simulink model "gridv1"  (R2021a)
settings: Solver=VariableStepAuto  StartTime=0.0  StopTime=inf  RelTol=1e-3
libraries: spsThreePhaseBreakerLib x12, spsMosfetLib x12, spsThreePhaseSeriesRLCLoadLib x10, spsMeanLib x6, pid_lib x5, simulink x4, spsPLL3phLib x4, spsThreePhaseVIMeasurementLib x4, spsAsynchronousMachineSIUnitsLib x2, spsDCVoltageSourceLib x2, spsFourierLib x2, spsGroundLib x2
(part 2 of 2)

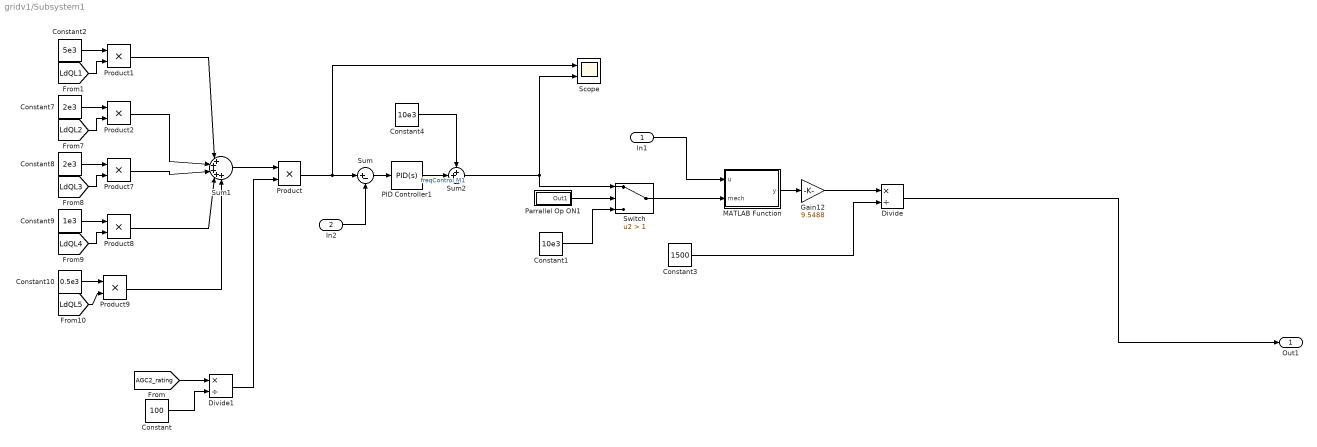
== system gridv1/Subsystem1 ==
  In1 : Inport
  In2 : Inport  Port=2
  Constant : Constant  Value=100
  Constant1 : Constant  Value=10e3
  Constant10 : Constant  Value=0.5e3
  Constant2 : Constant  Value=5e3
  Constant3 : Constant  Value=1500
  Constant4 : Constant  Value=10e3
  Constant7 : Constant  Value=2e3
  Constant8 : Constant  Value=2e3
  Constant9 : Constant  Value=1e3
  Divide : Product  Inputs=*/
  Divide1 : Product  Inputs=*/  OutDataTypeStr=Inherit: Same as first input
  Gain12 : Gain  Gain=9.5488
  MATLAB Function : MATLAB Function  TreatAsAtomicUnit=on
  PID Controller1 : pid_lib/PID Controller  Controller=PID  Form=Parallel  TimeDomain=Continuous-time  UseExternalTs=off  SampleTime=-1  IntegratorMethod=Forward Euler  FilterMethod=Forward Euler  ControllerParametersSource=internal  P=0.04  I=0.1  D=0  UseFilter=on  N=100  TunerSelectOption=Transfer Function Based (PID Tuner App)  ZeroCross=off  InitialConditionSource=internal  InitialConditionForIntegrator=0  InitialConditionForFilter=0  DifferentiatorICPrevScaledInput=0  ExternalReset=none  TrackingMode=off  Kt=1  LimitOutput=on  SatLimitsSource=internal  UpperSaturationLimit=500  LowerSaturationLimit=-500  LinearizeAsGain=on  AntiWindupMode=back-calculation  Kb=1  POutMin=[]  POutMax=[]  IOutMin=[]  IOutMax=[]  DOutMin=[]  DOutMax=[]  NOutMin=[]  NOutMax=[]  SumOutMin=[]  SumOutMax=[]  SaturationOutMin=[]  SaturationOutMax=[]  PParamMin=[]  PParamMax=[]  IParamMin=[]  IParamMax=[]  DParamMin=[]  DParamMax=[]  NParamMin=[]  NParamMax=[]  KbParamMin=[]  KbParamMax=[]  KtParamMin=[]  KtParamMax=[]  KbOutMin=[]  KbOutMax=[]  KtOutMin=[]  KtOutMax=[]  IntegratorOutMin=[]  IntegratorOutMax=[]  FilterOutMin=[]  FilterOutMax=[]  SumI1OutMin=[]  SumI1OutMax=[]  SumI2OutMin=[]  SumI2OutMax=[]  SumI3OutMin=[]  SumI3OutMax=[]  SumI4OutMin=[]  SumI4OutMax=[]  SumDOutMin=[]  SumDOutMax=[]  DifferentiatorOutMin=[]  DifferentiatorOutMax=[]  FilterDiffOutCoefMin=[]  FilterDiffOutCoefMax=[]  ReciprocalOutMin=[]  ReciprocalOutMax=[]  SumDenOutMin=[]  SumDenOutMax=[]  SumNumOutMin=[]  SumNumOutMax=[]  DivideOutMin=[]  DivideOutMax=[]  UdiffTsProdOutMin=[]  UdiffTsProdOutMax=[]  NTsProdOutMin=[]  NTsProdOutMax=[]  UintegralTsProdOutMin=[]  UintegralTsProdOutMax=[]  UngainTsProdOutMin=[]  UngainTsProdOutMax=[]  IntegratorContinuousStateAttributes=''  IntegratorStateMustResolveToSignalObject=off  IntegratorRTWStateStorageClass=Auto  FilterContinuousStateAttributes=''  FilterStateMustResolveToSignalObject=off  FilterRTWStateStorageClass=Auto  ParallelPVariant=InternalParameters  IdealPVariant=Disabled  IVariant=InternalParameters  DVariant=InternalParameters  IntegratorVariant=Continuous  SatVariant=Enabled  AWVariant=BackCalculation  PCopyVariant=Disabled  TRVariant=Disabled  FdbkBlocksVariant=Forward  IdealPFdbkVariant=Disabled  SatFdbkVariant=Disabled  DerivativeFilterVariant=ContFilter  NVariant=InternalParameters  NCopyVariant=Disabled  FilterICVariant=InternalICsFilter  IntegratorICVariant=InternalICs  ExternalResetVariant=Disabled  TRSumVariant=Passthrough  SumFdbkVariant=Disabled  SumVariant=Sum_PID  TsampFilterVariant=InternalTs  TsampNgainVariant=Passthrough  TsampIntegralVariant=Passthrough  ExternalSaturationOutDataTypeStr=Inherit: Same as second input
  Parrallel Op ON1 : Subsystem
  Product{,1..2,7..9} (6 alike) : Product  OutDataTypeStr=Inherit: Same as first input
  Scope : Scope  NumInputPorts=2
  Sum : Sum  Inputs=|+-
  Sum1 : Sum  Inputs=|+++++
  Sum2 : Sum  Inputs=++|
  Switch : Switch  Criteria=u2 > Threshold  Threshold=1
  Out1 : Outport
  wires:
  Gain12/1 -> Divide/1
  Divide/1 -> Out1/1
  Constant3/1 -> Divide/2
  MATLAB Function/1(y) -> Gain12/1
  In1/1 -> MATLAB Function/1(u)
  Switch/1 -> MATLAB Function/2(mech)
  Parrallel Op ON1/1(Out1) -> Switch/2
  Constant1/1 -> Switch/3
  Product9/1 -> Sum1/5
  Constant2/1 -> Product1/1
  Product7/1 -> Sum1/3
  Constant10/1 -> Product9/1
  Product8/1 -> Sum1/4
  Constant8/1 -> Product7/1
  Constant9/1 -> Product8/1
  [LdQL4] -> Product8/2
  Product1/1 -> Sum1/1
  [LdQL1] -> Product1/2
  Constant7/1 -> Product2/1
  Product2/1 -> Sum1/2
  [LdQL5] -> Product9/2
  [LdQL2] -> Product2/2
  [LdQL3] -> Product7/2
  In2/1 -> Sum/2
  Sum/1 -> PID Controller1/1
  [AGC2_rating] -> Divide1/1
  Constant/1 -> Divide1/2
  Divide1/1 -> Product/2
  Sum1/1 -> Product/1
  Product/1 -> Scope/1, Sum/1
  PID Controller1/1 -> Sum2/2  "freqControl M1"
  Constant4/1 -> Sum2/1
  Sum2/1 -> Scope/2, Switch/1

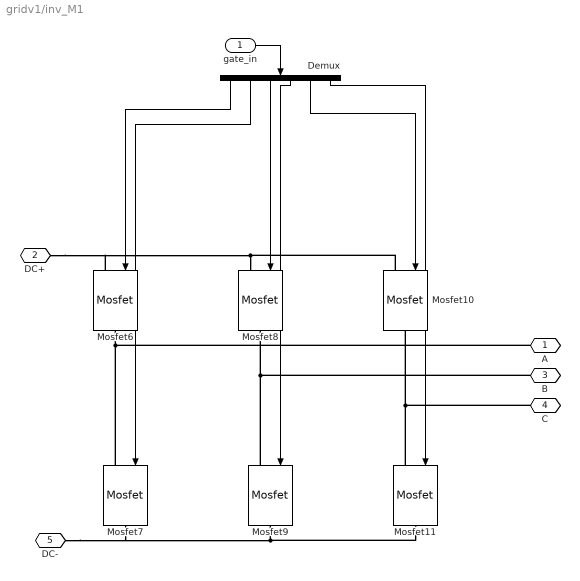
== system gridv1/inv_M1 ==
  gate_in : Inport
  Demux : Demux  Outputs=6
  Mosfet{6..11} (6 alike) : spsMosfetLib/Mosfet  Ron=0.1  Lon=0  Rd=0.01  Vfd=0  IC=0  Rs=1e5  Cs=inf  Measurements=off
  A : PMIOPort  Side=Right
  DC+ : PMIOPort  Port=2  Side=Left
  B : PMIOPort  Port=3  Side=Right
  C : PMIOPort  Port=4  Side=Right
  DC- : PMIOPort  Port=5  Side=Left
  wires:
  Demux/6 -> Mosfet11/1
  Demux/4 -> Mosfet9/1
  Demux/5 -> Mosfet10/1
  Demux/2 -> Mosfet7/1
  Demux/3 -> Mosfet8/1
  Demux/1 -> Mosfet6/1
  gate_in/1 -> Demux/1
  connections:
  Mosfet10/LConn1 -- DC+/RConn1 -- Mosfet6/LConn1 -- Mosfet8/LConn1
  Mosfet9/LConn1 -- B/RConn1 -- Mosfet8/RConn1
  Mosfet9/RConn1 -- DC-/RConn1 -- Mosfet7/RConn1 -- Mosfet11/RConn1
  Mosfet7/LConn1 -- A/RConn1 -- Mosfet6/RConn1
  Mosfet11/LConn1 -- C/RConn1 -- Mosfet10/RConn1

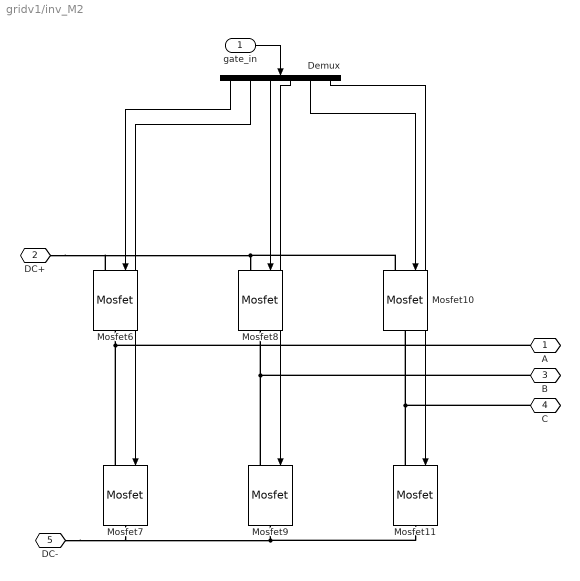
== system gridv1/inv_M2 ==
  gate_in : Inport
  Demux : Demux  Outputs=6
  Mosfet{6..11} (6 alike) : spsMosfetLib/Mosfet  Ron=0.1  Lon=0  Rd=0.01  Vfd=0  IC=0  Rs=1e5  Cs=inf  Measurements=off
  A : PMIOPort  Side=Right
  DC+ : PMIOPort  Port=2  Side=Left
  B : PMIOPort  Port=3  Side=Right
  C : PMIOPort  Port=4  Side=Right
  DC- : PMIOPort  Port=5  Side=Left
  wires:
  Demux/6 -> Mosfet11/1
  Demux/4 -> Mosfet9/1
  Demux/5 -> Mosfet10/1
  Demux/2 -> Mosfet7/1
  Demux/3 -> Mosfet8/1
  Demux/1 -> Mosfet6/1
  gate_in/1 -> Demux/1
  connections:
  Mosfet10/LConn1 -- DC+/RConn1 -- Mosfet6/LConn1 -- Mosfet8/LConn1
  Mosfet9/LConn1 -- B/RConn1 -- Mosfet8/RConn1
  Mosfet9/RConn1 -- DC-/RConn1 -- Mosfet7/RConn1 -- Mosfet11/RConn1
  Mosfet7/LConn1 -- A/RConn1 -- Mosfet6/RConn1
  Mosfet11/LConn1 -- C/RConn1 -- Mosfet10/RConn1

== system gridv1/Subsystem1/Parrallel Op ON1 ==
  Data Store Read : DataStoreRead  DataStoreName=synch1_  IndexOptions=Index vector (dialog)  Indices=1  OutputSizes=1
  Data Store Read1 : DataStoreRead  DataStoreName=synch2_  IndexOptions=Index vector (dialog)  Indices=1  OutputSizes=1
  Logical Operator : Logic  AllPortsSameDT=off  OutDataTypeStr=boolean
  Out1 : Outport
  wires:
  Data Store Read1/1 -> Logical Operator/2
  Logical Operator/1 -> Out1/1
  Data Store Read/1 -> Logical Operator/1

== matlab function gridv1/Relay_G2/MATLAB Function ==
  data: CBord input; rpm input; freq1 input; y output; sync1 input; sync2 input; sync output; delta_phase input
function [y,sync] = fcn(CBord, rpm, freq1, sync1, sync2, delta_phase)

if sync1 == 0 && sync2 == 0  
    if CBord == 1 && rpm > 1499.5 && freq1 > 49.5
        y = 1;
        sync = 1;
    else
        y = 0;
        sync = 0;
    end
elseif sync1 == 1 && sync2 == 0
    if delta_phase < 1 && CBord == 1 && rpm < 1500.5
        y = 1;
        sync = 1;
    else
        y = 0;
        sync = 0;
    end
else
    y = 1;
    sync = 1;
end

== matlab function gridv1/Relay_G1/MATLAB Function ==
  data: CBord input; rpm input; freq1 input; y output; sync1 input; sync2 input; sync output; delta_phase input
function [y,sync] = fcn(CBord, rpm, freq1, sync1, sync2, delta_phase)

if sync1 == 0 && sync2 == 0  
    if CBord == 1 && rpm > 1499.5 && freq1 > 49.5
        y = 1;
        sync = 1;
    else
        y = 0;
        sync = 0;
    end
elseif sync1 == 0 && sync2 == 1         
    if delta_phase < 1 && CBord == 1 && rpm < 1500.5
        y = 1;
        sync = 1;
    else
        y = 0;
        sync = 0;
    end
else
    y = 1;
    sync = 1;
end

== matlab function gridv1/MATLAB Function2 ==
  data: P1 input; Wm1 output; P2 input; P1ord input; P2ord input; CB input; userG1 input; userG2 input; Wm2 output; syncS input
function [Wm1, Wm2] = fcn(P1, P2, P1ord, P2ord, CB, userG1, userG2, syncS)

if syncS == 0 
    if (P1*1.05 < P1ord) && CB == 1
        Wm1 = 1500.2;
        Wm2 = 1500;
    elseif (P2*1.05 < P2ord) && CB == 1
        Wm1 = 1500;
        Wm2 = 1500.2;
    else
        Wm1 = userG1;
        Wm2 = userG2;
    end
else
    Wm1 = userG1;
    Wm2 = userG2;
end

== matlab function gridv1/Subsystem/MATLAB Function ==
  data: u input; y output; mech input
function y = fcn(u,mech)

if u < 52 && u > 48
    y = mech;
else
    y = 1;
end

== matlab function gridv1/Subsystem1/MATLAB Function ==
  data: u input; y output; mech input
function y = fcn(u,mech)

if u < 52 && u > 48
    y = mech;
else
    y = 1;
end

== matlab function gridv1/Speed SynchronizerM2 (phase angle) ==
  data: sync1 input; sync2 input; u input; y output
function y = fcn(sync1, sync2, u)

    if sync1 == 1 && sync2 == 0 && u < 1500.5
        y = 0.38;
    else
        y = 0;
    end

== matlab function gridv1/Speed SynchronizerM1 (phase angle) ==
  data: sync1 input; sync2 input; u input; y output
function y = fcn(sync1, sync2, u)

    if sync1 == 0 && sync2 == 1 && u < 1500.5
        y = 0.38;
    else
        y = 0;
    end
